simulink model "IMPIANTO_INSTABILE_Kcr"  (R2021a)
settings: Solver=VariableStepAuto  StartTime=0.0  StopTime=10.0  RelTol=1e-3
values from neighbouring files (symbols this model uses):
  A = processo.A    [esercizio1.m]
  B = processo.B    [esercizio1.m]
  C = processo.C    [esercizio1.m]
  D = processo.D    [esercizio1.m]
  Kcr = margin(G)    [esercizio1.m]
settings Model: Creator=Giorgio  LastModifiedBy=Giorgio

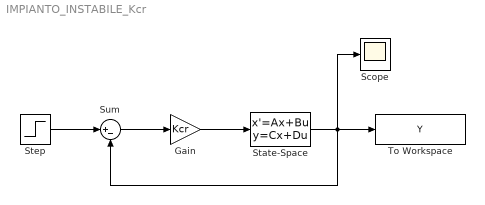
== system IMPIANTO_INSTABILE_Kcr ==
  Gain : Gain  Gain=Kcr
  Scope : Scope
  State-Space : StateSpace  A=A  B=B  C=C  D=D  InitialCondition=0
  Step : Step  Time=0  SampleTime=0
  Sum : Sum  Inputs=|+-
  To Workspace : ToWorkspace  VariableName=Y  SaveFormat=Timeseries  SampleTime=-1
  wires:
  Step/1 -> Sum/1
  Sum/1 -> Gain/1
  Gain/1 -> State-Space/1
  State-Space/1 -> Sum/2, Scope/1, To Workspace/1
